simulink model "closeloop_PI_Ga"  (R2022b)
settings: Solver=ode45  StartTime=0.0  StopTime=120  MaxStep=0.1  RelTol=1e-3  EnableMultiTasking=on
undefined symbols (not defined in the file): k1, k2, sigbuilder_block
settings Model: Creator=reza  LastModifiedBy=rezag
settings SolverCC: AlgebraicLoopSolver=TrustRegion
settings DataIOCC: LimitDataPoints=on  SaveFormat=Array  ReturnWorkspaceOutputs=off  OutputSaveName=Out1
settings OptimizationCC: LifeSpan=inf
settings DebuggingCC: SolverPrmCheckMsg=warning  UnconnectedInputMsg=warning  UnconnectedOutputMsg=warning  UnconnectedLineMsg=warning  SFUnexpectedBacktrackingDiag=warning  SFNoUnconditionalDefaultTransitionDiag=warning  SFExecutionAtInitializationDiag=none  SFMachineParentedDataDiag=warning  ArithmeticOperatorsInVariantConditions=warning
settings HardwareCC: ProdBitPerPointer=32  ProdBitPerSizeT=32  ProdBitPerPtrDiffT=32  ProdLargestAtomicFloat=None  ProdIntDivRoundTo=Undefined  ProdEndianess=Unspecified  ProdWordSize=32  ProdHWDeviceType=32-bit Generic
settings ModelReferenceCC: PropagateSignalLabelsOutOfModel=off
settings SFSimCC: SimUseLocalCustomCode=off  CustomCodeUndefinedFunction=UseInterfaceOnly
settings RTWCC: RTWUseLocalCustomCode=off
settings CodeAppCC: StateflowObjectComments=on
settings GRTTargetCC: TargetLangStandard=C89/C90 (ANSI)
settings ConfigComp: CovMetricSettings=dw  CovSaveCumulativeToWorkspaceVar=on  CovSaveSingleToWorkspaceVar=on  CovExternalEMLEnable=off  CovSFcnEnable=off

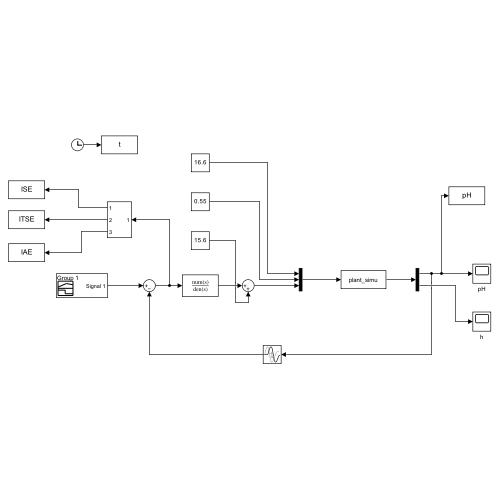
[thumbnail: Simulink's stored preview of the top-level diagram]
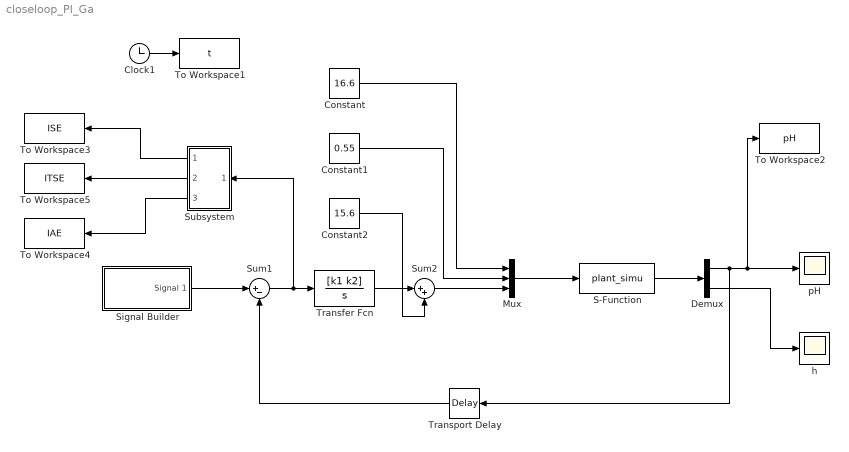
== system closeloop_PI_Ga ==
  Clock1 : Clock
  Constant : Constant  Value=16.6
  Constant1 : Constant  Value=0.55
  Constant2 : Constant  Value=15.6
  Demux : Demux  Outputs=2
  Mux : Mux  Inputs=3
  S-Function : S-Function  FunctionName=plant_simu  SFunctionDeploymentMode=off  EnableBusSupport=off
  Signal Builder : Subsystem  Tag=STV Subsys  LoadFcn=sigbuilder_block('load');  StartFcn=sigbuilder_block('start');  StopFcn=sigbuilder_block('stop');  ClipboardFcn=sigbuilder_block('clipboard');  mask(Sigbuilder block){tuvar=[0:10]}
      mask help: Simulink:masks:SigbuilderBlock_MD
      mask init:
      | if ~strcmp(get_param(bdroot(gcbh),'SimulationStatus'),'stopped') tuvar = sigbuilder_block('maskInit'); end
      settings: CopyFcn=sigbuilder_block('copy');  DeleteFcn=sigbuilder_block('delete');  ModelCloseFcn=sigbuilder_block('modelClose');  PreSaveFcn=sigbuilder_block('preSave');  PauseFcn=sigbuilder_block('pause');  ContinueFcn=sigbuilder_block('continue');  NameChangeFcn=sigbuilder_block('namechange');  OpenFcn=sigbuilder_block('open',[401.25 108 550.5 399.75 ]);  CloseFcn=sigbuilder_block('close');
      mask Display: plot(0, 0, 100, 100,[2, 2, 32, 32, 2], [68, 8, 8, 68, 68],[32, 2], [38, 38], [32, 19, 2],[53, 60, 44], [32, 17, 17, 2],[16, 16, 31, 31]);txt = getActiveGroup(gcbh);text(2, 100, txt,'verticalAlignment', 'top');
  Subsystem : Subsystem
  Sum1 : Sum  Inputs=|+-
  Sum2 : Sum  Inputs=|++
  To Workspace1 : ToWorkspace  VariableName=t  SaveFormat=Timeseries  SampleTime=-1
  To Workspace2 : ToWorkspace  VariableName=pH  SaveFormat=Timeseries  SampleTime=-1
  To Workspace3 : ToWorkspace  VariableName=ISE  SampleTime=-1
  To Workspace4 : ToWorkspace  VariableName=IAE  SampleTime=-1
  To Workspace5 : ToWorkspace  VariableName=ITSE  SampleTime=-1
  Transfer Fcn : TransferFcn  Numerator=[k1 k2]  Denominator=[1 0]
  Transport Delay : TransportDelay  DelayTime=0.167
  h : Scope
  pH : Scope
  wires:
  S-Function/1 -> Demux/1
  Mux/1 -> S-Function/1
  Demux/1 -> To Workspace2/1, pH/1, Transport Delay/1
  Demux/2 -> h/1
  Transport Delay/1 -> Sum1/2
  Constant/1 -> Mux/1
  Constant1/1 -> Mux/2
  Sum2/1 -> Mux/3
  Clock1/1 -> To Workspace1/1
  Signal Builder/1(Signal 1) -> Sum1/1
  Constant2/1 -> Sum2/2
  Transfer Fcn/1 -> Sum2/1
  Sum1/1 -> Subsystem/1(In1), Transfer Fcn/1
  Subsystem/1(Out1) -> To Workspace3/1
  Subsystem/2(Out2) -> To Workspace5/1
  Subsystem/3(Out3) -> To Workspace4/1

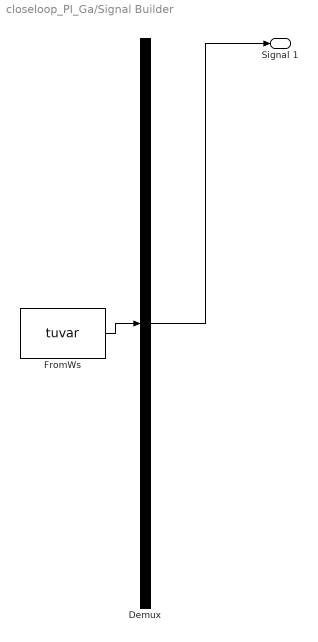
== system closeloop_PI_Ga/Signal Builder ==
  Demux : Demux  Tag=STV Demux  Outputs=1
      settings: DisplayOption=none
  FromWs : FromWorkspace  Tag=STV FromWs  VariableName=tuvar
      SigBuilderData=|
      | common.afterFinalStr = 'Extrapolate'
      | common.sampleTime = 0
      | dataSet.timeRange = [0 180]
      | dataSet.name = 'Group 1'
      | sbobj.Groups.Name = 'Group 1'
      | sbobj.Groups.Signals.Name = 'Signal 1'
      | sbobj.Groups.Signals.XData = [0 30 30 60 60 90 90 120 180]
      | sbobj.Groups.Signals.YData = [7 7 9 9 5 5 7 7 7]
      | sbobj.Groups.TimeRange = [0 180]
  Signal 1 : Outport  Tag=STV Outport
  wires:
  Demux/1 -> Signal 1/1
  FromWs/1 -> Demux/1

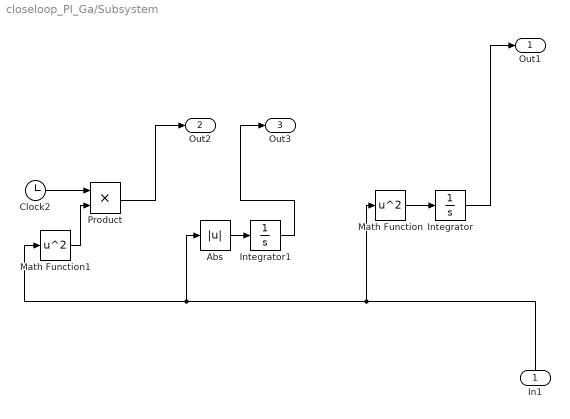
== system closeloop_PI_Ga/Subsystem ==
  In1 : Inport
  Abs : Abs  SaturateOnIntegerOverflow=off
  Clock2 : Clock
  Integrator : Integrator
  Integrator1 : Integrator
  Math Function : Math  Operator=square  SignedPower=on
  Math Function1 : Math  Operator=square  SignedPower=on
  Product : Product
  Out1 : Outport
  Out2 : Outport  Port=2
  Out3 : Outport  Port=3
  wires:
  Math Function/1 -> Integrator/1
  Abs/1 -> Integrator1/1
  Integrator/1 -> Out1/1
  Integrator1/1 -> Out3/1
  Clock2/1 -> Product/1
  In1/1 -> Math Function1/1, Abs/1, Math Function/1
  Math Function1/1 -> Product/2
  Product/1 -> Out2/1
